simulink model "robot2gdl"  (R2022a)
settings: Solver=ode4  StartTime=0.0  StopTime=2  FixedStep=0.0005  RelTol=1e-3
model workspace: external: MATLAB File G:\My Drive\WaveletDynamics Doctorado\Clases\Control de robots\Matlab\robot2gdl_simscape\robot2gdl_DataFile.m (data not in the file)
undefined symbols (not defined in the file or in its folder): smiData, X, Y, Z
libraries: sm_lib x15, nesl_utility x3
settings Model: Creator=benja  LastModifiedBy=benja

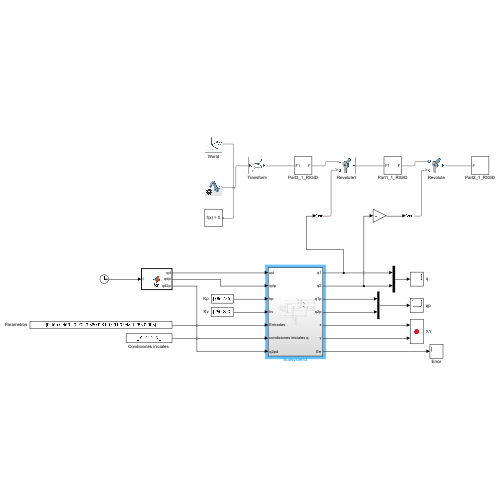
[thumbnail: Simulink's stored preview of the top-level diagram]
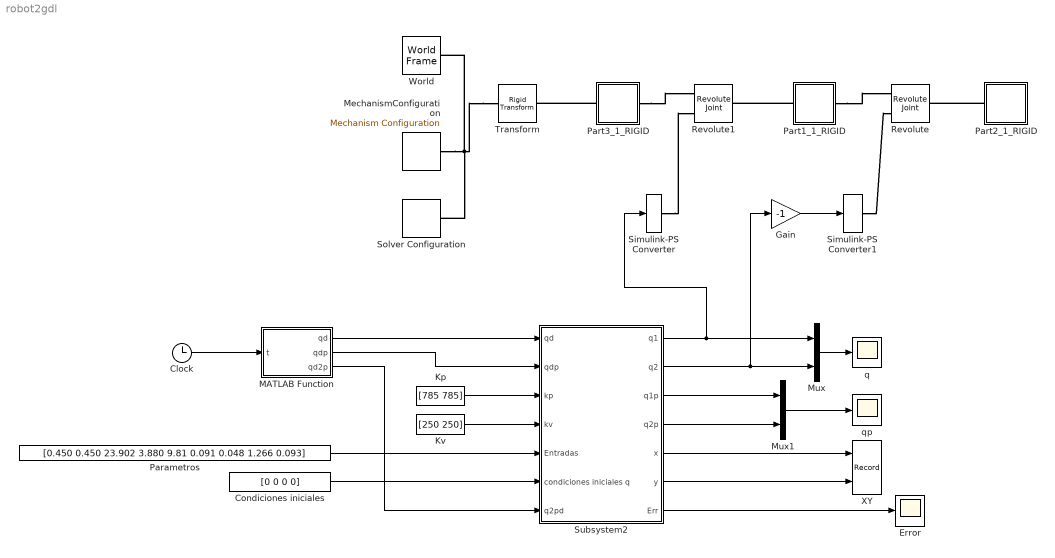
== system robot2gdl ==
  Clock : Clock
  "Condiciones iniciales " : Constant  Value=[0 0 0 0]
  Error : Scope
  Gain : Gain  Gain=-1
  Kp : Constant  Value=[785 785]
  Kv : Constant  Value=[250 250]
  MATLAB Function : MATLAB Function  TreatAsAtomicUnit=on
  MechanismConfiguration : sm_lib/Utilities/Mechanism Configuration  UniformGravity=Constant  GravityVector=[0 -9.80665 0]  GravityUnits=m/s^2  LinearizationDelta=0.001  JointModeTransitionNonlinearIterations=2
  Mux : Mux  Inputs=2
  Mux1 : Mux  Inputs=2
  Parametros : Constant  Value=[0.450 0.450 23.902 3.880 9.81 0.091 0.048 1.266 0.093]
  Part1_1_RIGID : Subsystem
  Part2_1_RIGID : Subsystem
  Part3_1_RIGID : Subsystem
  Revolute : sm_lib/Joints/Revolute Joint  JointMode=Normal  SenseConstraintForce=off  SenseConstraintForceX=off  SenseConstraintForceY=off  SenseConstraintForceZ=off  SenseConstraintTorque=off  SenseConstraintTorqueX=off  SenseConstraintTorqueY=off  SenseConstraintTorqueZ=off  SenseTotalForce=off  SenseTotalForceX=off  SenseTotalForceY=off  SenseTotalForceZ=off  SenseTotalTorque=off  SenseTotalTorqueX=off  SenseTotalTorqueY=off  SenseTotalTorqueZ=off  CompositeWrenchDir=FollowerOnBase  CompositeWrenchFrame=FollowerFrame  EquilibriumPosition=0  EquilibriumPositionUnits=deg  SpringStiffness=0  SpringStiffnessUnits=N*m/deg  DampingCoefficient=0  DampingCoefficientUnits=N*m/(deg/s)  TorqueActuationMode=ComputedTorque  MotionActuationMode=InputMotion  SensePosition=off  SenseVelocity=off  SenseAcceleration=off  SenseTorqueForce=off  SenseLowerLimitTorqueForce=off  SenseUpperLimitTorqueForce=off  LowerLimitSpecify=off  LowerLimitBound=-90  LowerLimitBoundUnits=deg  LowerLimitStiffness=1e4  LowerLimitStiffnessUnits=N*m/deg  LowerLimitDamping=10  LowerLimitDampingUnits=N*m/(deg/s)  LowerLimitTransitionRegionWidth=0.1  LowerLimitTransitionRegionWidthUnits=deg  UpperLimitSpecify=off  UpperLimitBound=90  UpperLimitBoundUnits=deg  UpperLimitStiffness=1e4  UpperLimitStiffnessUnits=N*m/deg  UpperLimitDamping=10  UpperLimitDampingUnits=N*m/(deg/s)  UpperLimitTransitionRegionWidth=0.1  UpperLimitTransitionRegionWidthUnits=deg  PositionTargetSpecify=on  PositionTargetPriority=Low  PositionTargetValue=smiData.RevoluteJoint(1).Rz.Pos  PositionTargetValueUnits=deg  VelocityTargetSpecify=off  VelocityTargetPriority=High  VelocityTargetValue=0  VelocityTargetValueUnits=deg/s
  Revolute1 : sm_lib/Joints/Revolute Joint  JointMode=Normal  SenseConstraintForce=off  SenseConstraintForceX=off  SenseConstraintForceY=off  SenseConstraintForceZ=off  SenseConstraintTorque=off  SenseConstraintTorqueX=off  SenseConstraintTorqueY=off  SenseConstraintTorqueZ=off  SenseTotalForce=off  SenseTotalForceX=off  SenseTotalForceY=off  SenseTotalForceZ=off  SenseTotalTorque=off  SenseTotalTorqueX=off  SenseTotalTorqueY=off  SenseTotalTorqueZ=off  CompositeWrenchDir=FollowerOnBase  CompositeWrenchFrame=BaseFrame  EquilibriumPosition=0  EquilibriumPositionUnits=deg  SpringStiffness=0  SpringStiffnessUnits=N*m/deg  DampingCoefficient=0  DampingCoefficientUnits=N*m/(deg/s)  TorqueActuationMode=ComputedTorque  MotionActuationMode=InputMotion  SensePosition=off  SenseVelocity=off  SenseAcceleration=off  SenseTorqueForce=off  SenseLowerLimitTorqueForce=off  SenseUpperLimitTorqueForce=off  LowerLimitSpecify=off  LowerLimitBound=-90  LowerLimitBoundUnits=deg  LowerLimitStiffness=1e4  LowerLimitStiffnessUnits=N*m/deg  LowerLimitDamping=10  LowerLimitDampingUnits=N*m/(deg/s)  LowerLimitTransitionRegionWidth=0.1  LowerLimitTransitionRegionWidthUnits=deg  UpperLimitSpecify=off  UpperLimitBound=90  UpperLimitBoundUnits=deg  UpperLimitStiffness=1e4  UpperLimitStiffnessUnits=N*m/deg  UpperLimitDamping=10  UpperLimitDampingUnits=N*m/(deg/s)  UpperLimitTransitionRegionWidth=0.1  UpperLimitTransitionRegionWidthUnits=deg  PositionTargetSpecify=on  PositionTargetPriority=Low  PositionTargetValue=smiData.RevoluteJoint(2).Rz.Pos  PositionTargetValueUnits=deg  VelocityTargetSpecify=off  VelocityTargetPriority=High  VelocityTargetValue=0  VelocityTargetValueUnits=deg/s
  Simulink-PS Converter : nesl_utility/Simulink-PS Converter  PhysicalDomain=network_engine_domain  SubClassName=ps_input  LeftPortType=input  RightPortType=output  PseudoPeriodic=off  Frequencies=[]  NoiseDistribution=none  NoiseParameters=[]  Unit=1  AffineConversion=off  FilteringAndDerivatives=filter  SimscapeFilterOrder=2  InputFilterTimeConstant=0.001  UdotUserProvided=0
      settings: SourceProductBaseCode=SS,PW,VE
  Simulink-PS Converter1 : nesl_utility/Simulink-PS Converter  PhysicalDomain=network_engine_domain  SubClassName=ps_input  LeftPortType=input  RightPortType=output  PseudoPeriodic=off  Frequencies=[]  NoiseDistribution=none  NoiseParameters=[]  Unit=1  AffineConversion=off  FilteringAndDerivatives=filter  SimscapeFilterOrder=2  InputFilterTimeConstant=0.001  UdotUserProvided=0
      settings: SourceProductBaseCode=SS,PW,VE
  Solver Configuration : nesl_utility/Solver Configuration  PhysicalDomain=network_engine_domain  SubClassName=solver  LeftPortType=input  RightPortType=generic  Tones=[]  Harmonics=[]  SimulateNoise=off  Profile=off  UseLocalSampling=off  EnableSwitchedLinearOptims=on  FrequencyDomain=off  UseCCode=off  RelTol=0.001  AbsTol=0.001  MinStep=1e-09  ToWorkspace=off  RevertToSquareIcSolve=off  NumHomotopyIterations=100  PhasorMode=off  PhasorModeNumHarmonics=1  IndexReductionMethod=DerivativeReplacement  DoDC=off  ResidualTolerance=1e-09  UseLocalSolver=off  LocalSolverChoice=NE_BACKWARD_EULER_ADVANCER  LocalSolverSampleTime=0.001  DoFixedCost=off  MaxNonlinIter=3  MaxModeIter=2  ComputeImpulses=off  ImpulseIterations=2  LinearAlgebra=auto  LinearAlgebraNumThread=0  EquationFormulation=NE_TIME_EF  DelaysMemoryBudget=1024  AutomaticFiltering=on  FilteringTimeConstant=0.001  PartitionStorageMethod=AS_NEEDED  PartitionMemoryBudget=1024  PartitionMethod=ROBUST
      settings: SourceProductBaseCode=SS,PW,VE
  Subsystem2 : Subsystem
  Transform : sm_lib/Frames and Transforms/Rigid Transform  TranslationMethod=Cartesian  TranslationStandardOffset=0  TranslationLengthUnit=mm  TranslationStandardAxis=+Z  TranslationCartesianOffset=smiData.RigidTransform(5).translation  TranslationROffset=0  TranslationROffsetUnits=m  TranslationZOffset=0  TranslationZOffsetUnits=m  TranslationThetaOffset=0  TranslationThetaOffsetUnits=deg  RotationMethod=ArbitraryAxis  RotationAngleUnits=rad  RotationStandardAxis=+Z  RotationAngle=smiData.RigidTransform(5).angle  RotationArbitraryAxis=smiData.RigidTransform(5).axis  FollAlignAxisA=+X  BaseAlignAxisA=+Y  FollAlignAxisB=+Y  BaseAlignAxisB=+Z  RotationSequenceAxes=FollowerAxes  RotationSequence=XYX  RotationSequenceAngles=[0 0 0]  RotationSequenceAnglesUnits=deg  RotationMatrix=[1 0 0; 0 1 0; 0 0 1]
  World : sm_lib/Frames and Transforms/World Frame
  XY : Record  FileSettingsInternal="{\"entries\":[{\"content\":{\"excelSettings\":{\"content\":{},\"type\":\"Streamout.ExcelSettings\"}},\"type\":\"Streamout.FileSettingStorage\",\"uuid\":\"a6f36b09-9445-4890-9c93-af0a9eab5696\"}],\"packageUris\":[\"http://schema.mathworks.com/mf0/streamout_blocks/R2020a\"],\"version\":\"1.0\"}"  Layout=[1 1]  SignalsInternal="{\"entries\":[{\"content\":{\"signals\":[{\"content\":{\"blockPath\":[\"robot2gdl/XY\"],\"channel\":[],\"dimensions\":[1],\"domain\":\"robot2gdl/XY\",\"lineColor\":\"#a2142f\",\"plots\":[1],\"port\":1,\"sid\":[\"\"],\"signalID\":10427,\"signalName\":\"Subsystem2:5\"},\"type\":\"RecordBlkView.Signal\",\"uuid\":\"30b602e6-a53c-4094-bf3a-b6b60ad22952\"},{\"content\":{\"blockPath\":[\"robot2gdl/XY\"],\"channel\":[],\"dimensions\":[1],\"domain\":\"robot2gdl/XY\",\"lineColor\":\"#139fff\",\"plots\":[1],\"port\":2,\"sid\":[\"\"],\"signalID\":10431,\"signalName\":\"Subsystem2:6\"},\"type\":\"RecordBlkView.Signal\",\"uuid\":\"4b790ca9-d91a-4c1f-891e-f566b0ffab8b\"}]},\"type\":\"RecordBlkView.InputSignals\",\"uuid\":\"1502a7cf-7cc3-4dc5-9aef-b574025ab8ab\"}],\"packageUris\":[\"http://schema.mathworks.com/mf0/streamout_blocks/R2020a\"],\"version\":\"1.0\"}"  VisualizationBindings="{\"xyplotplugin\":{\"info\":[{\"series\":[{\"bindingParametersList\":[{\"parameter\":\"X-Axis\",\"signalID\":10427,\"signalName\":\"Subsystem2:5\"},{\"parameter\":\"Y-Axis\",\"signalID\":10431,\"signalName\":\"Subsystem2:6\"}],\"seriesID\":22677}],\"subplotID\":1}]}}"  CompatibilityTag=XY  st=-1
  q : Scope
  qp : Scope
  wires:
  "Condiciones iniciales "/1 -> Subsystem2/6(condiciones iniciales q)
  Subsystem2/5(x) -> XY/1
  Subsystem2/6(y) -> XY/2
  Subsystem2/7(Err) -> Error/1
  Mux/1 -> q/1
  Parametros/1 -> Subsystem2/5(Entradas)
  Mux1/1 -> qp/1
  Kp/1 -> Subsystem2/3(kp)
  Subsystem2/4(q2p) -> Mux1/2
  Subsystem2/3(q1p) -> Mux1/1
  Kv/1 -> Subsystem2/4(kv)
  MATLAB Function/1(qd) -> Subsystem2/1(qd)
  Subsystem2/1(q1) -> Mux/1, Simulink-PS Converter/1
  Subsystem2/2(q2) -> Gain/1, Mux/2
  Gain/1 -> Simulink-PS Converter1/1
  MATLAB Function/2(qdp) -> Subsystem2/2(qdp)
  MATLAB Function/3(qd2p) -> Subsystem2/7(q2pd)
  Clock/1 -> MATLAB Function/1(t)
  connections:
  Transform/LConn1 -- MechanismConfiguration/RConn1 -- Solver Configuration/RConn1 -- World/RConn1
  Part1_1_RIGID/RConn1 -- Revolute/LConn1
  Part2_1_RIGID/LConn1 -- Revolute/RConn1
  Part3_1_RIGID/RConn1 -- Revolute1/LConn1
  Part1_1_RIGID/LConn1 -- Revolute1/RConn1
  Part3_1_RIGID/LConn1 -- Transform/RConn1
  Simulink-PS Converter/RConn1 -- Revolute1/LConn2
  Simulink-PS Converter1/RConn1 -- Revolute/LConn2

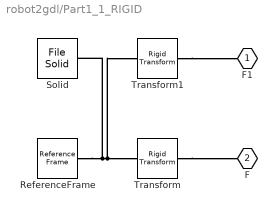
== system robot2gdl/Part1_1_RIGID ==
  ReferenceFrame : sm_lib/Frames and Transforms/Reference Frame
  Solid : sm_lib/Body Elements/File Solid  ExtGeomFileName=Part1_Default_sldprt.STL  UnitType=Custom  ExtGeomFileUnits=mm  StepReaderType=HEX  ExportConvexHullGeometry=off  InertiaType=Custom  Mass=smiData.Solid(2).mass  MassUnits=kg  CenterOfMass=smiData.Solid(2).CoM  CenterOfMassUnits=mm  MomentsOfInertia=smiData.Solid(2).MoI  MomentsOfInertiaUnits=kg*mm^2  ProductsOfInertia=smiData.Solid(2).PoI  ProductsOfInertiaUnits=kg*mm^2  BasedOnType=DensityFromFile  Density=1000  DensityUnits=kg/m^3  DoExposeReferenceFrame=on  SerializedFrames=<Frames/>  GraphicType=FromGeometry  MarkerShape=Sphere  MarkerSize=10  GraphicVisPropType=SimpleVisualProperties  GraphicDiffuseColor=smiData.Solid(2).color  GraphicSpecularColor=[0.5 0.5 0.5 1.0]  GraphicAmbientColor=[0.15 0.15 0.15 1.0]  GraphicEmissiveColor=[0.0 0.0 0.0 1.0]  GraphicShininess=75  GraphicOpacity=smiData.Solid(2).opacity
  Transform : sm_lib/Frames and Transforms/Rigid Transform  TranslationMethod=Cartesian  TranslationStandardOffset=0  TranslationLengthUnit=mm  TranslationStandardAxis=+Z  TranslationCartesianOffset=smiData.RigidTransform(1).translation  TranslationROffset=0  TranslationROffsetUnits=m  TranslationZOffset=0  TranslationZOffsetUnits=m  TranslationThetaOffset=0  TranslationThetaOffsetUnits=deg  RotationMethod=ArbitraryAxis  RotationAngleUnits=rad  RotationStandardAxis=+Z  RotationAngle=smiData.RigidTransform(1).angle  RotationArbitraryAxis=smiData.RigidTransform(1).axis  FollAlignAxisA=+X  BaseAlignAxisA=+Y  FollAlignAxisB=+Y  BaseAlignAxisB=+Z  RotationSequenceAxes=FollowerAxes  RotationSequence=XYX  RotationSequenceAngles=[0 0 0]  RotationSequenceAnglesUnits=deg  RotationMatrix=[1 0 0; 0 1 0; 0 0 1]
  Transform1 : sm_lib/Frames and Transforms/Rigid Transform  TranslationMethod=Cartesian  TranslationStandardOffset=0  TranslationLengthUnit=mm  TranslationStandardAxis=+Z  TranslationCartesianOffset=smiData.RigidTransform(4).translation  TranslationROffset=0  TranslationROffsetUnits=m  TranslationZOffset=0  TranslationZOffsetUnits=m  TranslationThetaOffset=0  TranslationThetaOffsetUnits=deg  RotationMethod=ArbitraryAxis  RotationAngleUnits=rad  RotationStandardAxis=+Z  RotationAngle=smiData.RigidTransform(4).angle  RotationArbitraryAxis=smiData.RigidTransform(4).axis  FollAlignAxisA=+X  BaseAlignAxisA=+Y  FollAlignAxisB=+Y  BaseAlignAxisB=+Z  RotationSequenceAxes=FollowerAxes  RotationSequence=XYX  RotationSequenceAngles=[0 0 0]  RotationSequenceAnglesUnits=deg  RotationMatrix=[1 0 0; 0 1 0; 0 0 1]
  F1 : PMIOPort  Side=Left
  F : PMIOPort  Port=2  Side=Right
  connections:
  Solid/RConn1 -- ReferenceFrame/RConn1 -- Transform/LConn1 -- Transform1/LConn1
  Transform/RConn1 -- F/RConn1
  Transform1/RConn1 -- F1/RConn1

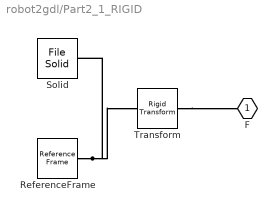
== system robot2gdl/Part2_1_RIGID ==
  ReferenceFrame : sm_lib/Frames and Transforms/Reference Frame
  Solid : sm_lib/Body Elements/File Solid  ExtGeomFileName=Part2_Default_sldprt.STL  UnitType=Custom  ExtGeomFileUnits=mm  StepReaderType=HEX  ExportConvexHullGeometry=off  InertiaType=Custom  Mass=smiData.Solid(3).mass  MassUnits=kg  CenterOfMass=smiData.Solid(3).CoM  CenterOfMassUnits=mm  MomentsOfInertia=smiData.Solid(3).MoI  MomentsOfInertiaUnits=kg*mm^2  ProductsOfInertia=smiData.Solid(3).PoI  ProductsOfInertiaUnits=kg*mm^2  BasedOnType=DensityFromFile  Density=1000  DensityUnits=kg/m^3  DoExposeReferenceFrame=on  SerializedFrames=<Frames/>  GraphicType=FromGeometry  MarkerShape=Sphere  MarkerSize=10  GraphicVisPropType=SimpleVisualProperties  GraphicDiffuseColor=smiData.Solid(3).color  GraphicSpecularColor=[0.5 0.5 0.5 1.0]  GraphicAmbientColor=[0.15 0.15 0.15 1.0]  GraphicEmissiveColor=[0.0 0.0 0.0 1.0]  GraphicShininess=75  GraphicOpacity=smiData.Solid(3).opacity
  Transform : sm_lib/Frames and Transforms/Rigid Transform  TranslationMethod=Cartesian  TranslationStandardOffset=0  TranslationLengthUnit=mm  TranslationStandardAxis=+Z  TranslationCartesianOffset=smiData.RigidTransform(2).translation  TranslationROffset=0  TranslationROffsetUnits=m  TranslationZOffset=0  TranslationZOffsetUnits=m  TranslationThetaOffset=0  TranslationThetaOffsetUnits=deg  RotationMethod=ArbitraryAxis  RotationAngleUnits=rad  RotationStandardAxis=+Z  RotationAngle=smiData.RigidTransform(2).angle  RotationArbitraryAxis=smiData.RigidTransform(2).axis  FollAlignAxisA=+X  BaseAlignAxisA=+Y  FollAlignAxisB=+Y  BaseAlignAxisB=+Z  RotationSequenceAxes=FollowerAxes  RotationSequence=XYX  RotationSequenceAngles=[0 0 0]  RotationSequenceAnglesUnits=deg  RotationMatrix=[1 0 0; 0 1 0; 0 0 1]
  F : PMIOPort  Side=Left
  connections:
  Solid/RConn1 -- ReferenceFrame/RConn1 -- Transform/LConn1
  Transform/RConn1 -- F/RConn1

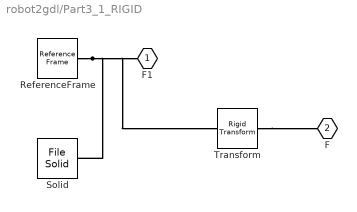
== system robot2gdl/Part3_1_RIGID ==
  ReferenceFrame : sm_lib/Frames and Transforms/Reference Frame
  Solid : sm_lib/Body Elements/File Solid  ExtGeomFileName=Part3_Default_sldprt.STL  UnitType=Custom  ExtGeomFileUnits=mm  StepReaderType=HEX  ExportConvexHullGeometry=off  InertiaType=Custom  Mass=smiData.Solid(1).mass  MassUnits=kg  CenterOfMass=smiData.Solid(1).CoM  CenterOfMassUnits=mm  MomentsOfInertia=smiData.Solid(1).MoI  MomentsOfInertiaUnits=kg*mm^2  ProductsOfInertia=smiData.Solid(1).PoI  ProductsOfInertiaUnits=kg*mm^2  BasedOnType=DensityFromFile  Density=1000  DensityUnits=kg/m^3  DoExposeReferenceFrame=on  SerializedFrames=<Frames/>  GraphicType=FromGeometry  MarkerShape=Sphere  MarkerSize=10  GraphicVisPropType=SimpleVisualProperties  GraphicDiffuseColor=smiData.Solid(1).color  GraphicSpecularColor=[0.5 0.5 0.5 1.0]  GraphicAmbientColor=[0.15 0.15 0.15 1.0]  GraphicEmissiveColor=[0.0 0.0 0.0 1.0]  GraphicShininess=75  GraphicOpacity=smiData.Solid(1).opacity
  Transform : sm_lib/Frames and Transforms/Rigid Transform  TranslationMethod=Cartesian  TranslationStandardOffset=0  TranslationLengthUnit=mm  TranslationStandardAxis=+Z  TranslationCartesianOffset=smiData.RigidTransform(3).translation  TranslationROffset=0  TranslationROffsetUnits=m  TranslationZOffset=0  TranslationZOffsetUnits=m  TranslationThetaOffset=0  TranslationThetaOffsetUnits=deg  RotationMethod=ArbitraryAxis  RotationAngleUnits=rad  RotationStandardAxis=+Z  RotationAngle=smiData.RigidTransform(3).angle  RotationArbitraryAxis=smiData.RigidTransform(3).axis  FollAlignAxisA=+X  BaseAlignAxisA=+Y  FollAlignAxisB=+Y  BaseAlignAxisB=+Z  RotationSequenceAxes=FollowerAxes  RotationSequence=XYX  RotationSequenceAngles=[0 0 0]  RotationSequenceAnglesUnits=deg  RotationMatrix=[1 0 0; 0 1 0; 0 0 1]
  F1 : PMIOPort  Side=Left
  F : PMIOPort  Port=2  Side=Right
  connections:
  Solid/RConn1 -- ReferenceFrame/RConn1 -- Transform/LConn1 -- F1/RConn1
  Transform/RConn1 -- F/RConn1

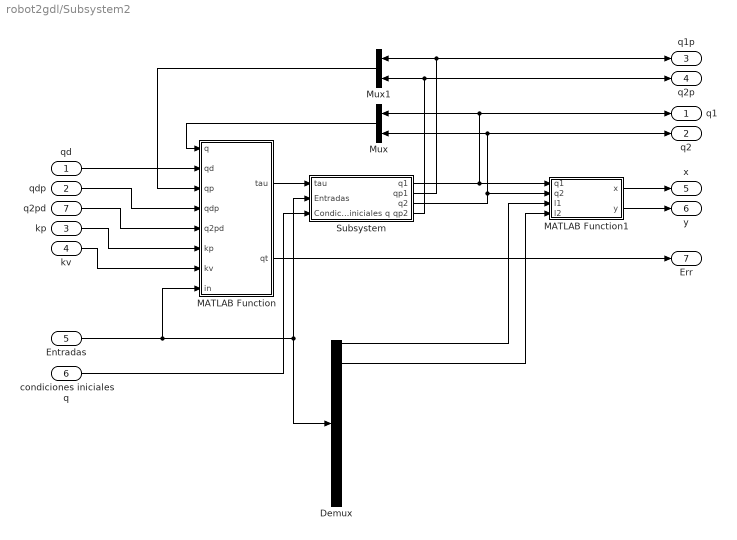
== system robot2gdl/Subsystem2 ==
  qd : Inport
  qdp : Inport  Port=2
  kp : Inport  Port=3
  kv : Inport  Port=4
  Entradas : Inport  Port=5
  condiciones iniciales q : Inport  Port=6
  q2pd : Inport  Port=7
  Demux : Demux  Outputs=9
  MATLAB Function : MATLAB Function  TreatAsAtomicUnit=on
  MATLAB Function1 : MATLAB Function  TreatAsAtomicUnit=on
  Mux : Mux  Inputs=2
  Mux1 : Mux  Inputs=2
  Subsystem : Subsystem
  q1 : Outport
  q2 : Outport  Port=2
  q1p : Outport  Port=3
  q2p : Outport  Port=4
  x : Outport  Port=5
  y : Outport  Port=6
  Err : Outport  Port=7
  wires:
  qdp/1 -> MATLAB Function/4(qdp)
  MATLAB Function/1(tau) -> Subsystem/1(tau)
  Mux1/1 -> MATLAB Function/3(qp)
  MATLAB Function/2(qt) -> Err/1
  Subsystem/2(qp1) -> q1p/1, Mux1/1
  Mux/1 -> MATLAB Function/1(q)
  Subsystem/3(q2) -> Mux/2, q2/1, MATLAB Function1/2(q2)
  qd/1 -> MATLAB Function/2(qd)
  Subsystem/1(q1) -> Mux/1, q1/1, MATLAB Function1/1(q1)
  Subsystem/4(qp2) -> Mux1/2, q2p/1
  MATLAB Function1/1(x) -> x/1
  MATLAB Function1/2(y) -> y/1
  kp/1 -> MATLAB Function/6(kp)
  kv/1 -> MATLAB Function/7(kv)
  Entradas/1 -> MATLAB Function/8(in), Subsystem/2(Entradas), Demux/1
  condiciones iniciales q/1 -> Subsystem/3(Condiciones iniciales q)
  q2pd/1 -> MATLAB Function/5(q2pd)
  Demux/1 -> MATLAB Function1/3(l1)
  Demux/2 -> MATLAB Function1/4(l2)

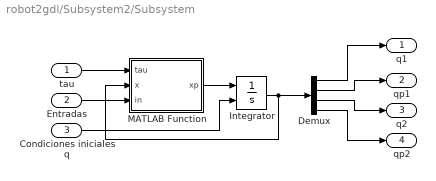
== system robot2gdl/Subsystem2/Subsystem ==
  tau : Inport
  Entradas : Inport  Port=2
  Condiciones iniciales q : Inport  Port=3
  Demux : Demux
  Integrator : Integrator  InitialConditionSource=external  InitialCondition=[0 0 0 0]
  MATLAB Function : MATLAB Function  TreatAsAtomicUnit=on
  q1 : Outport
  qp1 : Outport  Port=2
  q2 : Outport  Port=3
  qp2 : Outport  Port=4
  wires:
  MATLAB Function/1(xp) -> Integrator/1
  Demux/1 -> q1/1
  tau/1 -> MATLAB Function/1(tau)
  Demux/4 -> qp2/1
  Integrator/1 -> Demux/1, MATLAB Function/2(x)
  Demux/2 -> qp1/1
  Demux/3 -> q2/1
  Entradas/1 -> MATLAB Function/3(in)
  Condiciones iniciales q/1 -> Integrator/2

== matlab function robot2gdl/MATLAB Function ==
  data: t input; qd output; qdp output; qd2p output
function [qd, qdp, qd2p] = fcn(t)

a1 = pi/45;
b1 = pi/4;
c1 = pi/18;
w1 = 15;

a2 = pi/180;
b2 = pi/3;
c2 = (25*pi)/36;
w2 = 3.5;

qd1 = a1 + b1*(1 - exp(-2.0*t^3)) + c1*(1 - exp(-2.0*t^3))*sin(w1*t);
qd2 = a2 + b2*(1 - exp(-1.8*t^3)) + c2*(1 - exp(-1.8*t^3))*sin(w2*t);

qd = [qd1 qd2];

qdp1 = 6 * b1*t^(2)*exp(-2.0*t^3) + 6 * c1*t^(2)*exp(-2.0*t^3)*sin(w1*t) + (c1 - c1*exp(-2.0*t^3))*cos(w1*t)*w1;
qdp2 = 5.4*b2*t^(2)*exp(-1.8*t^3) + 5.4*c2*t^(2)*exp(-1.8*t^3)*sin(w2*t) + (c2 - c2*exp(-1.8*t^3))*cos(w2*t)*w2;

qdp = [qdp1 qdp2];

qd2p1 = 12 * b1*t*exp(-2.0*t^3) - 36 * b1*t^4*exp(-2.0*t^3) + 12 * c1*t*exp(-2.0*t^3)*sin(w1*t) - 36 * c1*t^4*exp(-2.0*t^3)*sin(w1*t) + 12 * c1*t^2*exp(-2.0*t^3)*cos(w1*t)*w1 - (c1-c1*exp(-2.0*t^3))*sin(w1*t)*w1^2;
qd2p2 = 10.8*b2*t*exp(-1.8*t^3) - 29.2*b2*t^4*exp(-1.8*t^3) + 10.8*c2*t*exp(-1.8*t^3)*sin(w2*t) - 29.2*c2*t^4*exp(-1.8*t^3)*sin(w2*t) + 10.8*c2*t^2*exp(-1.8*t^3)*cos(w2*t)*w2 - (c2-c2*exp(-1.8*t^3))*sin(w2*t)*w2^2;

qd2p = [qd2p1 qd2p2];

== matlab function robot2gdl/Subsystem2/MATLAB Function ==
  settings: updateMethod=DISCRETE
  data: q input; tau output; qd input; qp input; qdp input; q2pd input; kp input; kv input; qt output; in input
function [tau,qt]  = fcn(q,qd,qp,qdp,q2pd,kp,kv,in)

l1  = in(1); % m
l2  = in(2); % m
m1  = in(3); % kg
m2  = in(4); % kg
g   = in(5);
lc1 = in(6); % m
lc2 = in(7); % m
I1  = in(8); %kg m^2
I2  = in(9); %kg m^2


qt1 = qd(1) - q(1);
qt2 = qd(2) - q(2);

qtp1 = qdp(1) - qp(1);
qtp2 = qdp(2) - qp(2);

qt = [qt1 qt2];

qtp = [qtp1 qtp2];

x = [q(1) qp(1) q(2) qp(2)];

%%%%%%%%%%%%%%%%%%%%%%%%%%%%%%%%%%%%%%%%%%%%%%%%%%%%%%%%%%%%%%%%%%%%%%%%%%%
m = [m1 m2];
lc = [lc1 lc2];
l = [l1 l2];
I = [I1 I2];

M11 = m(1)*lc(1)^2 + m(2)*(l(1)^2 + lc(2)^2 + 2*l(1)*lc(2)*cos(x(3))) + I(1) + I(2);
M12 = m(2)*(lc(2)^2 + l(1)*lc(2)*cos(x(3))) + I(2);
M21 = m(2)*(lc(2)^2 + l(1)*lc(2)*cos(x(3))) + I(2);
M22 = m(2)*lc(2)^2 + I(2);

M = [M11 M12; M21 M22];

C11 = -m(2)*l(1)*lc(2)*sin(x(3))*x(4);
C12 = -m(2)*l(1)*lc(2)*sin(x(3))*(x(2)+x(4));
C21 = m(2)*l(1)*lc(2)*sin(x(3))*x(2);
C22 = 0;

C = [C11 C12; C21 C22]; 


g1 = (m1*lc1 + m2*l1)*g*sin(x(1)) + m2*lc2*g*sin(x(1)+x(3));
g2 = m2*lc2*g*sin(x(1) + x(3));
%%%%%%%%%%%%%%%%%%%%%%%%%%%%%%%%%%%%%%%%%%%%%%%%%%%%%%%%%%%%%%%%%%%%%%%%%%% 


tau1 = kp(1)*qt(1) + kv(1)*qtp(1) + (M11*q2pd(1) + M12*q2pd(2)) + (C11*qdp(1) + C12*qdp(2)) + g1;
tau2 = kp(2)*qt(2) + kv(2)*qtp(2) + (M21*q2pd(1) + M22*q2pd(2)) + (C21*qdp(1) + C22*qdp(2)) + g2;


tau = [tau1 tau2];

== matlab function robot2gdl/Subsystem2/MATLAB Function1 ==
  data: q1 input; x output; q2 input; y output; l1 input; l2 input
function [x,y] = fcn(q1, q2, l1, l2)
% l1 = 0.1933; % m
% l2 = 0.1458; % m
l = [l1 l2];
q = [q1 q2];
x = l(1)*sin(q(1)) + l(2)*sin(q(1) + q(2));
y = -l(1)*cos(q(1)) - l(2)*cos(q(1) + q(2));

== matlab function robot2gdl/Subsystem2/Subsystem/MATLAB Function ==
  data: tau input; xp output; x input; in input
function xp = fcn(tau,x,in)

l1  = in(1); % m
l2  = in(2); % m
m1  = in(3); % kg
m2  = in(4); % kg
g   = in(5);
lc1 = in(6); % m
lc2 = in(7); % m
I1  = in(8); %kg m^2
I2  = in(9); %kg m^2


m = [m1 m2];
lc = [lc1 lc2];
l = [l1 l2];
I = [I1 I2];

%%%%%%%%%%%%%%%%%%%%%%%%%%%%%%%%%%%%%%%%%%%%%%%%%%%%%%%%%%%%%%%%%%%%%%%%%%%
m = [m1 m2];
lc = [lc1 lc2];
l = [l1 l2];
I = [I1 I2];

M11 = m(1)*lc(1)^2 + m(2)*(l(1)^2 + lc(2)^2 + 2*l(1)*lc(2)*cos(x(3))) + I(1) + I(2);
M12 = m(2)*(lc(2)^2 + l(1)*lc(2)*cos(x(3))) + I(2);
M21 = m(2)*(lc(2)^2 + l(1)*lc(2)*cos(x(3))) + I(2);
M22 = m(2)*lc(2)^2 + I(2);

M = [M11 M12; M21 M22];

C11 = -m(2)*l(1)*lc(2)*sin(x(3))*x(4);
C12 = -m(2)*l(1)*lc(2)*sin(x(3))*(x(2)+x(4));
C21 = m(2)*l(1)*lc(2)*sin(x(3))*x(2);
C22 = 0;

C = [C11 C12; C21 C22]; 


g1 = (m1*lc1 + m2*l1)*g*sin(x(1)) + m2*lc2*g*sin(x(1)+x(3));
g2 = m2*lc2*g*sin(x(1) + x(3));
%%%%%%%%%%%%%%%%%%%%%%%%%%%%%%%%%%%%%%%%%%%%%%%%%%%%%%%%%%%%%%%%%%%%%%%%%%% 

gV = [g1 g2]; 

D1 = M(1,1)*M(2,2)-M(1,2)*M(2,1);
D2 = tau(1)-C(1,1)*x(2)-C(1,2)*x(4)-gV(1);
D3 = tau(2)-C(2,1)*x(2)-C(2,2)*x(4)-gV(2);

D4 = M(1,1)*M(2,2)-M(1,2)*M(2,1);
D5 = tau(1)-C(1,1)*x(2)-C(1,2)*x(4)-gV(1);
D6 = tau(2)-C(2,1)*x(2)-C(2,2)*x(4)-gV(2);

x1p = x(2);
x2p = (M(2,2)*D5-M(1,2)*D6)/D4;
x3p = x(4);
x4p = (-M(2,1)*D5+M(1,1)*D6)/D4;

q2p1 = (1/D1)*(M(2,2)*D2-M(1,2)*D3);
q2p2 = (1/D1)*(-M(2,1)*D2+M(1,1)*D3);

q2p = [q2p1 q2p2];

xp = [x1p x2p x3p x4p];
